simulink model "analysisModel"  (R2018b)
settings: Solver=ode45  StartTime=0.0  StopTime=10.0  RelTol=1e-3  EnableMultiTasking=on
values from neighbouring files (symbols this model uses):
  J = 0.5    [demo_hinf.m]
  K = ss(CL.Blocks.K0)    [demo_hinf.m]
settings Model: ExtModeAutoUpdateStatusClock=off  Creator=biannic  LastModifiedBy=croos
settings DataIOCC: LimitDataPoints=on  SaveFormat=Array  SignalLoggingSaveFormat=ModelDataLogs  SignalLoggingName=sigsOut
settings OptimizationCC: DefaultParameterBehavior=Inlined  BufferReuse=off  ExpressionDepthLimit=2147483647  LifeSpan=inf
settings DebuggingCC: SaveWithParameterizedLinksMsg=none  UnderspecifiedInitializationDetection=Classic  MergeDetectMultiDrivingBlocksExec=none  SignalResolutionControl=TryResolveAllWithWarning  MultiTaskDSMMsg=warning  MultiTaskCondExecSysMsg=none  StateNameClashWarn=warning  InitInArrayFormatMsg=none  SFUnexpectedBacktrackingDiag=warning  SFNoUnconditionalDefaultTransitionDiag=warning  SFExecutionAtInitializationDiag=none
settings HardwareCC: ProdBitPerPointer=32  ProdBitPerSizeT=32  ProdBitPerPtrDiffT=32  ProdLargestAtomicFloat=None  ProdIntDivRoundTo=Undefined  ProdEndianess=Unspecified  ProdWordSize=32  ProdHWDeviceType=32-bit Generic  TargetUnknown=on
settings ModelReferenceCC: PropagateSignalLabelsOutOfModel=off
settings SFSimCC: SimUseLocalCustomCode=off
settings RTWCC: RTWUseLocalCustomCode=off
settings CodeAppCC: StateflowObjectComments=on
settings GRTTargetCC: TargetLangStandard=C89/C90 (ANSI)  GeneratePreprocessorConditionals=Disable all  CombineOutputUpdateFcns=off  GRTInterface=on
settings ConfigComp: CovMetricSettings=dw  CovHtmlReporting=on  CovSaveCumulativeToWorkspaceVar=on  CovSaveSingleToWorkspaceVar=on  CovExternalEMLEnable=off  CovSFcnEnable=off

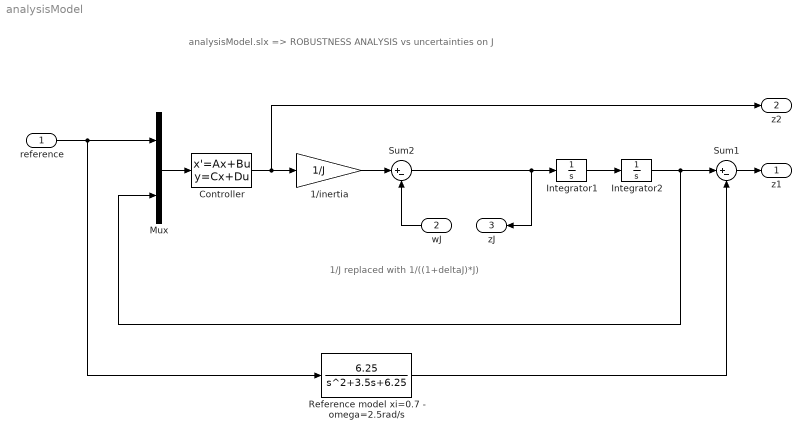
== system analysisModel ==
  note: 1/J replaced with 1/((1+deltaJ)*J)
  note: analysisModel.slx => ROBUSTNESS ANALYSIS vs uncertainties on J
  reference : Inport
  wJ : Inport  Port=2
  1/inertia : Gain  Gain=1/J  SaturateOnIntegerOverflow=on  OutDataTypeStr=Inherit: Same as input  ParamDataTypeStr=Inherit: Same as input
  Controller : StateSpace  A=K.a  B=K.b  C=K.c  D=K.d  InitialCondition=0
  Integrator1 : Integrator
  Integrator2 : Integrator
  Mux : Mux  Inputs=2
  Reference model xi=0.7 - omega=2.5rad/s : TransferFcn  Numerator=[6.25]  Denominator=[1 3.5 6.25]
  Sum1 : Sum  Inputs=|+-  SaturateOnIntegerOverflow=on
  Sum2 : Sum  Inputs=|+-  SaturateOnIntegerOverflow=on
  z1 : Outport  VectorParamsAs1DForOutWhenUnconnected=on
  z2 : Outport  Port=2  VectorParamsAs1DForOutWhenUnconnected=on
  zJ : Outport  Port=3  VectorParamsAs1DForOutWhenUnconnected=on
  wires:
  Integrator1/1 -> Integrator2/1
  Integrator2/1 -> Sum1/1, Mux/2
  reference/1 -> Mux/1, Reference model xi=0.7 - omega=2.5rad/s/1
  Controller/1 -> 1/inertia/1, z2/1
  Reference model xi=0.7 - omega=2.5rad/s/1 -> Sum1/2
  Sum1/1 -> z1/1
  Mux/1 -> Controller/1
  Sum2/1 -> Integrator1/1, zJ/1
  1/inertia/1 -> Sum2/1
  wJ/1 -> Sum2/2
